simulink model "Dynamic_RR"  (R2019b)
settings: Solver=VariableStepAuto  StartTime=0.0  StopTime=30  FixedStep=1e-2  RelTol=1e-3
values from neighbouring files (symbols this model uses):
  a = 0.0678    [define_vars.m]
  A = 0.9000    (= 0.9)    [define_vars.m]
  B = 1.0198    [define_vars.m]
  b = 0.1697    [define_vars.m]
  delta = 1.4642    [define_vars.m]
  pi_hat_0 = pi_param *(1+0.1)    [define_vars.m]
  pi_param = [1;0.333333333333333;1;0.333333333333333]    [define_vars.m]
  qInitial_0 = [1; 0.5]    [Initialization.m]    (also in define_vars.m = [1;1.2]')
settings Model: Creator=Stefano  LastModifiedBy=Stefano

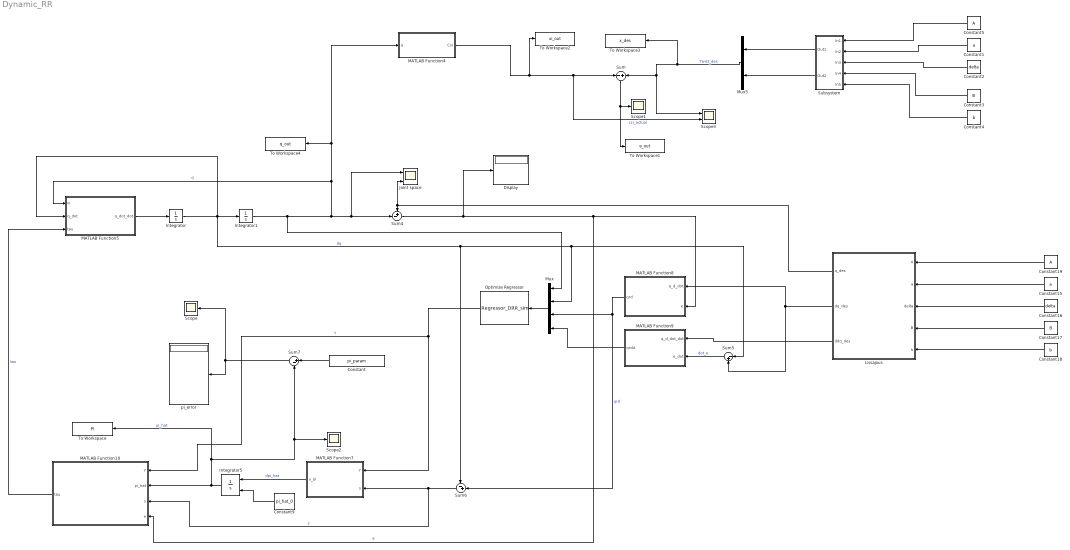
== system Dynamic_RR ==
  Constant : Constant  Value=pi_param
  Constant1 : Constant  Value=a
  Constant15 : Constant  Value=a
  Constant16 : Constant  Value=delta
  Constant17 : Constant  Value=B
  Constant18 : Constant  Value=b
  Constant19 : Constant  Value=A
  Constant2 : Constant  Value=delta
  Constant3 : Constant  Value=B
  Constant4 : Constant  Value=b
  Constant5 : Constant  Value=A
  Constant9 : Constant  Value=pi_hat_0
  Display : Display
  Integrator : Integrator  InitialCondition=qInitial_0
  Integrator1 : Integrator  InitialCondition=[0,0]'
  Integrator5 : Integrator  InitialConditionSource=external
  Joint space : Scope  NumInputPorts=2
  Lissajous : Subsystem
  MATLAB Function10 : MATLAB Function  TreatAsAtomicUnit=on
  MATLAB Function4 : MATLAB Function  TreatAsAtomicUnit=on
  MATLAB Function5 : MATLAB Function  TreatAsAtomicUnit=on
  MATLAB Function7 : MATLAB Function  TreatAsAtomicUnit=on
  MATLAB Function8 : MATLAB Function  TreatAsAtomicUnit=on
  MATLAB Function9 : MATLAB Function  TreatAsAtomicUnit=on
  Mux : Mux
  Mux5 : Mux  Inputs=2
  "Optimize Regressor " : MATLABFcn  MATLABFcn=Regressor_DRR_sim  OutputDimensions=[2,4]  Output1D=off
  Scope : Scope
  Scope1 : Scope
  Scope2 : Scope
  Scope3 : Scope  NumInputPorts=2
  Subsystem : Subsystem
  Sum : Sum  Inputs=-+
  Sum4 : Sum  Inputs=+-|
  Sum5 : Sum  Inputs=|-+
  Sum6 : Sum  Inputs=-+|
  Sum7 : Sum  Inputs=|+-
  To Workspace : ToWorkspace  VariableName=PI  SaveFormat=Timeseries  SampleTime=-1
  To Workspace1 : ToWorkspace  VariableName=e_out  SaveFormat=Timeseries  SampleTime=-1
  To Workspace2 : ToWorkspace  VariableName=xi_out  SaveFormat=Timeseries  SampleTime=-1
  To Workspace3 : ToWorkspace  VariableName=x_des  SaveFormat=Timeseries  SampleTime=-1
  To Workspace4 : ToWorkspace  VariableName=q_out  SaveFormat=Timeseries  SampleTime=-1
  pi_error : Display
  wires:
  Sum6/1 -> MATLAB Function10/3(s), MATLAB Function7/2(s)  "s"
  Sum4/1 -> Display/1, MATLAB Function10/4(e), MATLAB Function8/2(e)  "e"
  Sum5/1 -> MATLAB Function9/2(e_dot)  "dot_e"
  MATLAB Function7/1(u_pi) -> Integrator5/1  "dpi_hat"
  Integrator5/1 -> MATLAB Function10/2(pi_hat), To Workspace/1, Scope2/1, Sum7/2  "pi_hat"
  Integrator/1 -> MATLAB Function5/2(q_dot), Sum5/1, Mux/2, Sum6/1, Integrator1/1  "dq"
  Constant9/1 -> Integrator5/2
  MATLAB Function8/1(qrd) -> Sum6/2, Mux/3  "qrd"
  Mux/1 -> "Optimize Regressor "/1
  MATLAB Function9/1(qrdd) -> Mux/4
  Constant/1 -> Sum7/1
  Sum7/1 -> Scope/1, pi_error/1
  Integrator1/1 -> Mux/1, To Workspace4/1, MATLAB Function4/1(q), MATLAB Function5/1(q), Joint space/1, Sum4/2  "q"
  "Optimize Regressor "/1 -> MATLAB Function10/1(Y), MATLAB Function7/1(Y)  "Y"
  MATLAB Function10/1(tau) -> MATLAB Function5/3(tau)  "tau"
  MATLAB Function4/1(Csi) -> To Workspace2/1, Scope3/2, Sum/1  "csi_actual"
  Mux5/1 -> To Workspace3/1, Scope3/1, Sum/2  "Twist_des"
  Sum/1 -> To Workspace1/1, Scope1/1
  MATLAB Function5/1(q_dot_dot) -> Integrator/1
  Lissajous/1(q_des) -> Joint space/2, Sum4/1
  Lissajous/2(dq_des) -> MATLAB Function8/1(q_d_dot), Sum5/2
  Constant19/1 -> Lissajous/1(A)
  Constant15/1 -> Lissajous/2(a)
  Constant16/1 -> Lissajous/3("delta ")
  Constant17/1 -> Lissajous/4(B)
  Constant18/1 -> Lissajous/5(b)
  Lissajous/3(ddq_des) -> MATLAB Function9/1(q_d_dot_dot)
  Constant5/1 -> Subsystem/1(In1)
  Constant1/1 -> Subsystem/2(In2)
  Constant2/1 -> Subsystem/3(In3)
  Constant3/1 -> Subsystem/4(In4)
  Constant4/1 -> Subsystem/5(In5)
  Subsystem/1(Out1) -> Mux5/1
  Subsystem/2(Out2) -> Mux5/2

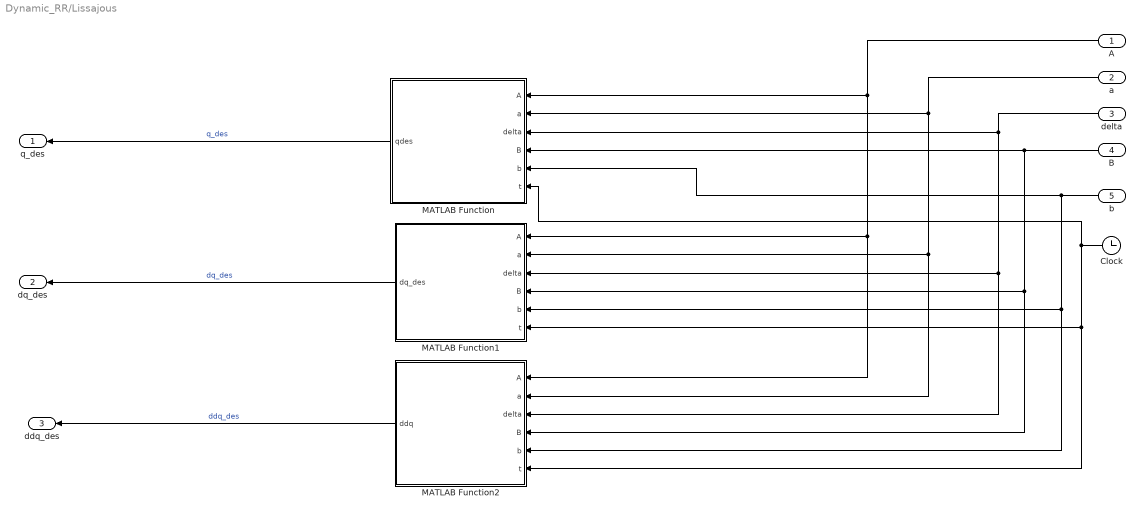
== system Dynamic_RR/Lissajous ==
  A : Inport
  a : Inport  Port=2
  "delta " : Inport  Port=3
  B : Inport  Port=4
  b : Inport  Port=5
  Clock : Clock
  MATLAB Function : MATLAB Function  TreatAsAtomicUnit=on
  MATLAB Function1 : MATLAB Function  TreatAsAtomicUnit=on
  MATLAB Function2 : MATLAB Function  TreatAsAtomicUnit=on
  q_des : Outport
  dq_des : Outport  Port=2
  ddq_des : Outport  Port=3
  wires:
  MATLAB Function1/1(dq_des) -> dq_des/1  "dq_des"
  MATLAB Function/1(qdes) -> q_des/1  "q_des"
  MATLAB Function2/1(ddq) -> ddq_des/1  "ddq_des"
  A/1 -> MATLAB Function2/1(A), MATLAB Function1/1(A), MATLAB Function/1(A)
  a/1 -> MATLAB Function2/2(a), MATLAB Function1/2(a), MATLAB Function/2(a)
  "delta "/1 -> MATLAB Function2/3(delta), MATLAB Function1/3(delta), MATLAB Function/3(delta)
  B/1 -> MATLAB Function1/4(B), MATLAB Function2/4(B), MATLAB Function/4(B)
  b/1 -> MATLAB Function1/5(b), MATLAB Function2/5(b), MATLAB Function/5(b)
  Clock/1 -> MATLAB Function2/6(t), MATLAB Function1/6(t), MATLAB Function/6(t)

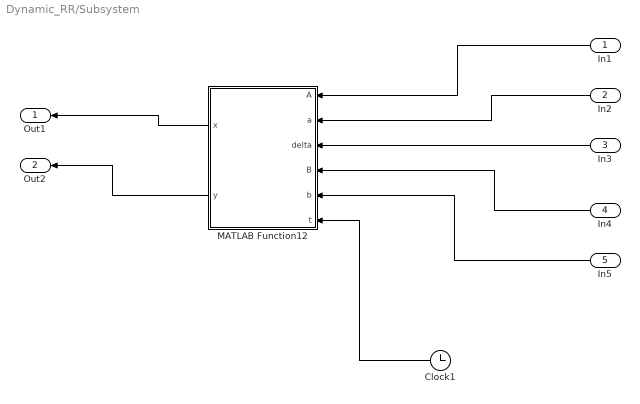
== system Dynamic_RR/Subsystem ==
  In1 : Inport
  In2 : Inport  Port=2
  In3 : Inport  Port=3
  In4 : Inport  Port=4
  In5 : Inport  Port=5
  Clock1 : Clock
  MATLAB Function12 : MATLAB Function  TreatAsAtomicUnit=on
  Out1 : Outport
  Out2 : Outport  Port=2
  wires:
  MATLAB Function12/1(x) -> Out1/1
  Clock1/1 -> MATLAB Function12/6(t)
  In5/1 -> MATLAB Function12/5(b)
  In2/1 -> MATLAB Function12/2(a)
  MATLAB Function12/2(y) -> Out2/1
  In3/1 -> MATLAB Function12/3(delta)
  In4/1 -> MATLAB Function12/4(B)
  In1/1 -> MATLAB Function12/1(A)

== matlab function Dynamic_RR/Lissajous/MATLAB Function1 ==
  data: A input; dq_des output; a input; delta input; B input; b input; t input
function dq_des = d_Lissajous(A,a,delta,B,b,t)


dq1 = ((a*cos(delta + a*t)*sin(delta + a*t)*A^2 + b*cos(b*t)*sin(b*t)*B^2)*(1 - ((B^2*sin(b*t)^2)/2 + (A^2*sin(delta + a*t)^2)/2 - 1)^2)^(1/2) + ((a*cos(delta + a*t)*sin(delta + a*t)*A^2 + b*cos(b*t)*sin(b*t)*B^2)*((B^2*sin(b*t)^2)/2 + (A^2*sin(delta + a*t)^2)/2)*((B^2*sin(b*t)^2)/2 + (A^2*sin(delta + a*t)^2)/2 - 1))/(1 - ((A^2*sin(delta + a*t)^2)/2 + (B^2*sin(b*t)^2)/2 - 1)^2)^(1/2))/(((B^2*sin(b*t)^2)/2 + (A^2*sin(delta + a*t)^2)/2)^2 - ((B^2*sin(b*t)^2)/2 + (A^2*sin(delta + a*t)^2)/2 - 1)^2 + 1) - (A*B*a*cos(delta + a*t)*sin(b*t) - A*B*b*sin(delta + a*t)*cos(b*t))/(A^2*sin(delta + a*t)^2 + B^2*sin(b*t)^2);

dq2 = - (a*cos(delta + a*t)*sin(delta + a*t)*A^2 + b*cos(b*t)*sin(b*t)*B^2)*(1 - ((B^2*sin(b*t)^2)/2 + (A^2*sin(delta + a*t)^2)/2 - 1)^2)^(1/2) - ((a*cos(delta + a*t)*sin(delta + a*t)*A^2 + b*cos(b*t)*sin(b*t)*B^2)*((B^2*sin(b*t)^2)/2 + (A^2*sin(delta + a*t)^2)/2 - 1)^2)/(1 - ((A^2*sin(delta + a*t)^2)/2 + (B^2*sin(b*t)^2)/2 - 1)^2)^(1/2);

dq_des = [dq1;dq2];

== matlab function Dynamic_RR/Lissajous/MATLAB Function ==
  data: A input; qdes output; a input; delta input; B input; b input; t input
function qdes = Lissajou(A,a,delta,B,b,t)

q1 = atan2(B*sin(b*t), A*sin(delta + a*t)) - atan2((4 - (A^2*sin(delta + a*t)^2 + B^2*sin(b*t)^2 - 2)^2)^(1/2)/2, (A^2*sin(delta + a*t)^2)/2 + (B^2*sin(b*t)^2)/2);
q2 = atan2((4 - (A^2*sin(delta + a*t)^2 + B^2*sin(b*t)^2 - 2)^2)^(1/2)/2, (A^2*sin(delta + a*t)^2)/2 + (B^2*sin(b*t)^2)/2 - 1);

qdes = [q1;q2];

== matlab function Dynamic_RR/Lissajous/MATLAB Function2 ==
  data: A input; ddq output; a input; delta input; B input; b input; t input
function ddq = dd_Lissajous(A,a,delta,B,b,t)

q1_ddot = (A*B*(a*sin(2*delta + 2*a*t)*A^2 + b*sin(2*b*t)*B^2)*(a*cos(delta + a*t)*sin(b*t) - b*sin(delta + a*t)*cos(b*t)))/(A^2*sin(delta + a*t)^2 + B^2*sin(b*t)^2)^2 - ((a*sin(2*delta + 2*a*t)*A^2 + b*sin(2*b*t)*B^2)*((a*sin(2*delta + 2*a*t)*A^2)/2 + (b*sin(2*b*t)*B^2)/2))/((A^2*sin(delta + a*t)^2 + B^2*sin(b*t)^2)*(4 - (A^2*sin(delta + a*t)^2 + B^2*sin(b*t)^2 - 2)^2)^(1/2)) - (B^6*b^2*(sin(b*t)^4 - 2*sin(b*t)^6) - B^4*b^2*sin(2*b*t)^2 - A^4*a^2*sin(2*delta + 2*a*t)^2 - 4*A^4*a^2*sin(delta + a*t)^2*cos(2*delta + 2*a*t) + A^6*a^2*sin(delta + a*t)^4*cos(2*delta + 2*a*t) + 2*B^4*b^2*cos(2*b*t)*(cos(2*b*t) - 1) - 4*A^2*B^2*a^2*sin(b*t)^2*cos(2*delta + 2*a*t) + A^2*B^4*a^2*sin(b*t)^4*cos(2*delta + 2*a*t) - 4*A^2*B^2*b^2*sin(delta + a*t)^2*cos(2*b*t) + A^4*B^2*b^2*sin(delta + a*t)^4*cos(2*b*t) + 2*A^2*B^4*b^2*sin(delta + a*t)^2*cos(2*b*t)*sin(b*t)^2 - 2*A^2*B^2*a*b*sin(2*b*t)*sin(2*delta + 2*a*t) + 2*A^4*B^2*a^2*sin(delta + a*t)^2*sin(b*t)^2*cos(2*delta + 2*a*t))/(4 - (A^2*sin(delta + a*t)^2 + B^2*sin(b*t)^2 - 2)^2)^(3/2) + (A*B*sin(delta + a*t)*sin(b*t)*(a^2 - b^2))/(A^2*sin(delta + a*t)^2 + B^2*sin(b*t)^2);

q2_ddot = - ((B^2*b^2*cos(2*b*t) + A^2*a^2*cos(2*delta + 2*a*t))*(4 - (A^2*sin(delta + a*t)^2 + B^2*sin(b*t)^2 - 2)^2)^(1/2))/2 - ((a*sin(2*delta + 2*a*t)*A^2 + b*sin(2*b*t)*B^2)^2*((B^2*sin(b*t)^2)/2 + (A^2*sin(delta + a*t)^2)/2 - 1))/(2*(4 - (A^2*sin(delta + a*t)^2 + B^2*sin(b*t)^2 - 2)^2)^(1/2)) - ((a*sin(2*delta + 2*a*t)*A^2 + b*sin(2*b*t)*B^2)^2*(A^2*sin(delta + a*t)^2 + B^2*sin(b*t)^2 - 2)^3)/(4*(4 - (A^2*sin(delta + a*t)^2 + B^2*sin(b*t)^2 - 2)^2)^(3/2)) - ((B^2*b^2*cos(2*b*t) + A^2*a^2*cos(2*delta + 2*a*t))*(A^2*sin(delta + a*t)^2 + B^2*sin(b*t)^2 - 2)^2)/(2*(4 - (A^2*sin(delta + a*t)^2 + B^2*sin(b*t)^2 - 2)^2)^(1/2));

ddq = [q1_ddot; q2_ddot];

== matlab function Dynamic_RR/MATLAB Function5 ==
  data: q input; q_dot_dot output; q_dot input; tau input
function q_dot_dot = Forward_Dynamics(q,q_dot,tau)

m1 = 1;
m2 = 1;

l1=1;
l2=1;

r1=l1/2;
r2=l2/2;


Izz1 = (1/12)*m1*l1^2;
Izz2 = (1/12)*m2*l2^2;



Alpha = Izz1 + Izz2 + m1*(r1)^2 + m2*(l1^2+r2^2);
Beta = m2*l1*r2;
Delta = Izz2 +m2*r2^2;

M = [Alpha + 2* Beta *cos(q(2)), Delta + Beta *cos(q(2));
     Delta + Beta *cos(q(2)),    Delta];

C = [-Beta*sin(q(2))*q_dot(2), -Beta*sin(q(2))*(q_dot(1)+q_dot(2));
     Beta*sin(q(2))*q_dot(1),   0];



q_dot_dot = inv(M)*([tau(1); tau(2)]- C*[q_dot(1); q_dot(2)]);

== matlab function Dynamic_RR/Subsystem/MATLAB Function12 ==
  data: x output; A input; y output; a input; delta input; B input; b input; t input
function [x,y] = Lissajous(A,a,delta,B,b,t)


x = A*sin(a*t+delta);
y = B*sin(b*t);


end

== matlab function Dynamic_RR/MATLAB Function4 ==
  data: q input; Csi output
function Csi  = Direct_Kinematics_RR(q)

%INPUT: q(1) = q1;
%       q(2) = q2;

%OUTPUT: px = position along x axis
%        py = position along y axis

%Link's lenght

l1 = 1;
l2 = 1;

px = l1 * cos(q(1)) + l2 * cos(q(1)+q(2));
py = l1 * sin(q(1)) + l2 * sin(q(1)+q(2));

Csi = [px; py];
end

== matlab function Dynamic_RR/MATLAB Function10 ==
  data: Y input; tau output; pi_hat input; s input; e input
function tau = Back_Stepping_Control_Law(Y,pi_hat,s,e)

Kd = 10 * eye(2);
Kp = 10 * eye(2);

tau = Y * pi_hat + Kd * s + Kp * e;

end

== matlab function Dynamic_RR/MATLAB Function7 ==
  data: Y input; u_pi output; s input
function u_pi = Update_Law(Y,s)

R = eye(2,4);
u_pi = pinv(R).*(Y.')*s;
end

== matlab function Dynamic_RR/MATLAB Function8 ==
  data: q_d_dot input; qrd output; e input
function qrd = q_r_dot(q_d_dot,e)

lambda = 7  * eye(2);
qrd = q_d_dot + lambda * e;

end

== matlab function Dynamic_RR/MATLAB Function9 ==
  data: q_d_dot_dot input; qrdd output; e_dot input
function qrdd = q_r_dot_dot(q_d_dot_dot,e_dot)

lambda = 7 * eye(2);
qrdd = q_d_dot_dot + lambda*e_dot;

end
